simulink library "LibEEPROM_eeprom_example_ORIGINAL"  (Simulink 10.0)
settings: Solver=VariableStepAuto  StartTime=0.0  StopTime=10.0  RelTol=1e-3
undefined symbols (not defined in the file): CRC32_calc_and_EEPROM_Write_ALL, crc32_calc_intern, CRC32_EEPROM_Read, EEPROM_Mirror, EEPROM_Read, IO_Blk_Lib_TTC500, IO_EEPROM_GetStatus, IO_EEPROM_Init, IO_EEPROM_Write, Read_Mirror, Write_Mirror, Write_Mirror_prepare_EEPROM
libraries: simulink x56
(part 1 of 8)
settings Model: Creator=hokka  LastModifiedBy=hokka

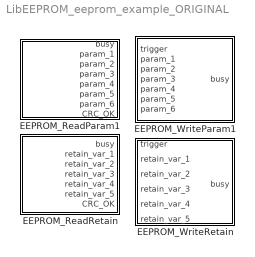
== system LibEEPROM_eeprom_example_ORIGINAL ==
  EEPROM_ReadParam1 : Subsystem  Priority=0  mask(Generated EEPROM_Read){}
      mask help: This Block was generated by the EEPROM Importer
      mask Help:
      | Read out the EEPROM for all given parameters and provide these values on the outports.
      | Reading is done at startup. As long as reading form EEPROM is not terminated for all parameters the busy flag will stay 'true'.
      | CRC_OK will be 0 as long as reading of EEPROM is not completed. Upon success the result is +1. If CRC check fails the result will be -1.
  EEPROM_ReadRetain : Subsystem  Priority=0  mask(Generated EEPROM_Read){}
      mask help: This Block was generated by the EEPROM Importer
      mask Help:
      | Read out the EEPROM for all given parameters and provide these values on the outports.
      | Reading is done at startup. As long as reading form EEPROM is not terminated for all parameters the busy flag will stay 'true'.
      | CRC_OK will be 0 as long as reading of EEPROM is not completed. Upon success the result is +1. If CRC check fails the result will be -1.
  EEPROM_WriteParam1 : Subsystem  Priority=0  mask(Generated EEPROM_Write){}
      mask help: This Block was generated by the EEPROM Importer
      mask Help:
      | Aufter receiving the positive edge of a trigger signal the EEPROM_Write - Block will store the parameters into the EEPROM together with the updated CRC32.
      | The busy flag will be 'true' as long as writing to EEPROM is not accomplished or any other EEPROM access is ongoing.
      | The busy flag needs not to be fed back as the trigger rise an internal pending activity as long as EEPROM is not accessible in order to accomplishe the actual writing as soon as the EEPROM is accessible again.
  EEPROM_WriteRetain : Subsystem  Priority=0  mask(Generated EEPROM_Write){}
      mask help: This Block was generated by the EEPROM Importer
      mask Help:
      | Aufter receiving the positive edge of a trigger signal the EEPROM_Write - Block will store the parameters into the EEPROM together with the updated CRC32.
      | The busy flag will be 'true' as long as writing to EEPROM is not accomplished or any other EEPROM access is ongoing.
      | The busy flag needs not to be fed back as the trigger rise an internal pending activity as long as EEPROM is not accessible in order to accomplishe the actual writing as soon as the EEPROM is accessible again.

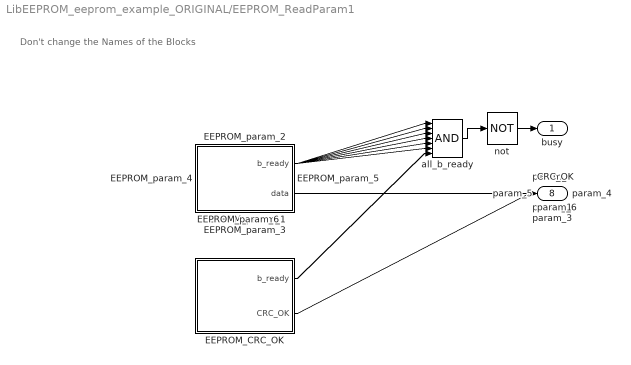
== system LibEEPROM_eeprom_example_ORIGINAL/EEPROM_ReadParam1 ==
  note: Don't change the Names of the Blocks
  EEPROM_CRC_OK : Subsystem  LoadFcn=|  mask(CRC32_EEPROM_Read_Code){SampleTime=-1, ttlib=IO_Blk_Lib_TTC500, ttDescription=CRC32_EEPROM_Read, tt_iolib_version=0.26, BasicAddr=4096, EndAddr=4110, offset=4111, length=4}
      | try
      | %
      | %Upgrade Information - standard BEGIN
      | new_color = 'blue';
      | new_ver = '0.26';
      | act_ver = get_param(gcb,'tt_iolib_version');
      | if not(strcmp(act_ver,new_ver))
      |     disp(['Upgrade block: ',gcb,char(10),'       Version: ',act_ver,' to ',new_ver]);
      |     %switch - case for specific upgrade information e.g. additional parameter required 
      |     %Change appearance and version information
      |     set_param(gcb,'ForegroundColor',new_color);
      |     set_param(gcb,'tt_iolib_version',new_ver);
      | end
      | %Upgrade Information - standard END
      | catch
      | %Standard catch section BEGIN
      | errordlg('An error occurred in a callback of the TTC580-BlockLib. Please open the Diagnostic Viewer for further details');
      | disp(' ');
      | disp('------------------------------------------------------------');
      | disp('An error occurred in a callback of the TTC580-BlockLib.');
      | disp(['Please check the parameters in the mask of ',gcb]);
      | disp('If you do not encounter any violations, then please '); 
      | disp('copy the following lines and report this to support@ttcontrol.com ');
      | disp('<< begin of error message dump >>');
      | disp(['Version of TTC580-BlockLib: ', get_param(gcb,'tt_iolib_version')]);
      | disp(get_param(gcb,'ttDescription'));
      | disp(gcb);
      | x=lasterror;disp(x.message);
      | disp(get_param(gcb,'MaskValues'));
      | disp(version);
      | disp(computer);
      | disp('<< end of error message dump >>');
      | disp('------------------------------------------------------------');
      | disp(' ');
      | %Standard catch section END
      | end
      mask help:
      | Calculate crc32 for the section [BasicAddr .. EndAddr] out of the EEPROM and compare to the content of a given address (=offset) in EEPROM.
      | The output CRC_OK may hold three possible values:
      | -1 => after EEPROM section was read, CRC check failed (terminal state)
      |   0 => reading of EEPROM section not completed yet, CRC check is pending
      | +1 => after EEPROM section was read, CRC check was successful (terminal state)
      mask init:
      | try
      | %%CT>
      | TAG_loc = get_param(gcb,'Tag');
      | if ~isempty(TAG_loc),[~,y]=regexp(TAG_loc,'(^[a-zA-Z0-9_]*)');
      |     if isempty(y) || y~=builtin('length',(TAG_loc)) %don't use length() alone!
      |         error(['The Tag: ',TAG_loc,' needs to start with a letter and may only contain the characters 0-9,a-Z,_ .']);
      | end,end
      | x=find_system(gcbh,'FollowLinks','on','LookUnderMasks','on','BlockType','S-Function');
      | for i=1:builtin('length',(x)) %don't use length() alone!
      |     set_param(x(i),'Tag',TAG_loc);
      | end
      | %<CT%
      | 
      | catch
      | %Standard catch section BEGIN
      | errordlg('An error occurred in a callback of the TTC580-BlockLib. Please open the Diagnostic Viewer for further details');
      | disp(' ');
      | disp('------------------------------------------------------------');
      | disp('An error occurred in a callback of the TTC580-BlockLib.');
      | disp(['Please check the parameters in the mask of ',gcb]);
      | disp('If you do not encounter any violations, then please '); 
      | disp('copy the following lines and report this to support@ttcontrol.com ');
      | disp('<< begin of error message dump >>');
      | disp(['Version of TTC580-BlockLib: ', get_param(gcb,'tt_iolib_version')]);
      | disp(get_param(gcb,'ttDescription'));
      | disp(gcb);
      | x=lasterror;disp(x.message);
      | disp(get_param(gcb,'MaskValues'));
      | disp(version);
      | disp(computer);
      | disp('<< end of error message dump >>');
      | disp('------------------------------------------------------------');
      | disp(' ');
      | %Standard catch section END
      | end
      settings: CopyFcn=%deleted
      mask Callback BasicAddr: %
      mask Callback EndAddr: %
      mask Callback offset: %
      mask Callback length: %
  EEPROM_param_1 : Subsystem  LoadFcn=|  mask(EEPROM_Read_Code){SampleTime=-1, ttlib=IO_Blk_Lib_TTC500, ttDescription=EEPROM_Read, tt_iolib_version=0.26, offset=4096, EEPROM_type=uint16}
      | try
      | %
      | %Upgrade Information - standard BEGIN
      | new_color = 'blue';
      | new_ver = '0.26';
      | act_ver = get_param(gcb,'tt_iolib_version');
      | if not(strcmp(act_ver,new_ver))
      |     disp(['Upgrade block: ',gcb,char(10),'       Version: ',act_ver,' to ',new_ver]);
      |     %switch - case for specific upgrade information e.g. additional parameter required 
      |     %Change appearance and version information
      |     set_param(gcb,'ForegroundColor',new_color);
      |     set_param(gcb,'tt_iolib_version',new_ver);
      | end
      | %Upgrade Information - standard END
      | catch
      | %Standard catch section BEGIN
      | errordlg('An error occurred in a callback of the TTC580-BlockLib. Please open the Diagnostic Viewer for further details');
      | disp(' ');
      | disp('------------------------------------------------------------');
      | disp('An error occurred in a callback of the TTC580-BlockLib.');
      | disp(['Please check the parameters in the mask of ',gcb]);
      | disp('If you do not encounter any violations, then please '); 
      | disp('copy the following lines and report this to support@ttcontrol.com ');
      | disp('<< begin of error message dump >>');
      | disp(['Version of TTC580-BlockLib: ', get_param(gcb,'tt_iolib_version')]);
      | disp(get_param(gcb,'ttDescription'));
      | disp(gcb);
      | x=lasterror;disp(x.message);
      | disp(get_param(gcb,'MaskValues'));
      | disp(version);
      | disp(computer);
      | disp('<< end of error message dump >>');
      | disp('------------------------------------------------------------');
      | disp(' ');
      | %Standard catch section END
      | end
      mask help:
      | Read data from the EEPROM.
      | Note that offset has to be in the range (0..65535 bytes)
      mask init:
      | try
      | switch EEPROM_type 
      |     case {'uint8'}
      |         length = 1; 
      |     case {'uint16'}; 
      |         length = 2; 
      |     case {'uint32'}
      |         length = 4; 
      |     case {'int8'}
      |         length = 1; 
      |     case {'int16'}; 
      |         length = 2; 
      |     case {'int32'}
      |         length = 4; 
      |     case {'single'}
      |         length = 4; 
      |     case {'double'}
      |         length = 8; 
      |     otherwise
      |         error('EEPROM_Read: unsupported type');
      | end
      | %%CT>
      | TAG_loc = get_param(gcb,'Tag');
      | if ~isempty(TAG_loc),[~,y]=regexp(TAG_loc,'(^[a-zA-Z0-9_]*)');
      |     if isempty(y) || y~=builtin('length',(TAG_loc)) %don't use length() alone!
      |         error(['The Tag: ',TAG_loc,' needs to start with a letter and may only contain the characters 0-9,a-Z,_ .']);
      | end,end
      | x=find_system(gcbh,'FollowLinks','on','LookUnderMasks','on','BlockType','S-Function');
      | for i=1:builtin('length',(x)) %don't use length() alone!
      |     set_param(x(i),'Tag',TAG_loc);
      | end
      | %<CT%
      | 
      | catch
      | %Standard catch section BEGIN
      | errordlg('An error occurred in a callback of the TTC580-BlockLib. Please open the Diagnostic Viewer for further details');
      | disp(' ');
      | disp('------------------------------------------------------------');
      | disp('An error occurred in a callback of the TTC580-BlockLib.');
      | disp(['Please check the parameters in the mask of ',gcb]);
      | disp('If you do not encounter any violations, then please '); 
      | disp('copy the following lines and report this to support@ttcontrol.com ');
      | disp('<< begin of error message dump >>');
      | disp(['Version of TTC580-BlockLib: ', get_param(gcb,'tt_iolib_version')]);
      | disp(get_param(gcb,'ttDescription'));
      | disp(gcb);
      | x=lasterror;disp(x.message);
      | disp(get_param(gcb,'MaskValues'));
      | disp(version);
      | disp(computer);
      | disp('<< end of error message dump >>');
      | disp('------------------------------------------------------------');
      | disp(' ');
      | %Standard catch section END
      | end
      settings: CopyFcn=%deleted
      mask Help: Parameter:<br>offset: [0..65535] place in the EEPROM where data shall be retieved from.<br>EEPROM_type: defines the length of data to be read from EEPROM. Possible values: uint8 (=1byte), uint16 (=2bytes), uint32 (=4bytes).<br><br>Output:<br>b_ready: when reading from EEPROM is not accomplished the output is FALSE.<br>data: Actual value that was retrieved from EEPROM.<br><br>Note: When the expression (offset + length) of Bytes exceed the limit of 65535 no  reading from EEPROM takes place and a constant zero is output as data and b_ready is FALSE.<br>When b_ready is not TRUE do not trust data as reading of EEPROM is not finished at startup of the ECU.<br><br>
      mask Callback offset: %
      mask TypeOptions EEPROM_type: uint8 | uint16 | uint32
      mask Callback EEPROM_type: %
  EEPROM_param_2 : Subsystem  LoadFcn=|  mask(EEPROM_Read_Code){SampleTime=-1, ttlib=IO_Blk_Lib_TTC500, ttDescription=EEPROM_Read, tt_iolib_version=0.26, offset=4098, EEPROM_type=uint16}
      | try
      | %
      | %Upgrade Information - standard BEGIN
      | new_color = 'blue';
      | new_ver = '0.26';
      | act_ver = get_param(gcb,'tt_iolib_version');
      | if not(strcmp(act_ver,new_ver))
      |     disp(['Upgrade block: ',gcb,char(10),'       Version: ',act_ver,' to ',new_ver]);
      |     %switch - case for specific upgrade information e.g. additional parameter required 
      |     %Change appearance and version information
      |     set_param(gcb,'ForegroundColor',new_color);
      |     set_param(gcb,'tt_iolib_version',new_ver);
      | end
      | %Upgrade Information - standard END
      | catch
      | %Standard catch section BEGIN
      | errordlg('An error occurred in a callback of the TTC580-BlockLib. Please open the Diagnostic Viewer for further details');
      | disp(' ');
      | disp('------------------------------------------------------------');
      | disp('An error occurred in a callback of the TTC580-BlockLib.');
      | disp(['Please check the parameters in the mask of ',gcb]);
      | disp('If you do not encounter any violations, then please '); 
      | disp('copy the following lines and report this to support@ttcontrol.com ');
      | disp('<< begin of error message dump >>');
      | disp(['Version of TTC580-BlockLib: ', get_param(gcb,'tt_iolib_version')]);
      | disp(get_param(gcb,'ttDescription'));
      | disp(gcb);
      | x=lasterror;disp(x.message);
      | disp(get_param(gcb,'MaskValues'));
      | disp(version);
      | disp(computer);
      | disp('<< end of error message dump >>');
      | disp('------------------------------------------------------------');
      | disp(' ');
      | %Standard catch section END
      | end
      mask help:
      | Read data from the EEPROM.
      | Note that offset has to be in the range (0..65535 bytes)
      mask init: same as LibEEPROM_eeprom_example_ORIGINAL/EEPROM_ReadParam1/EEPROM_param_1
      settings: CopyFcn=%deleted
      mask Help: Parameter:<br>offset: [0..65535] place in the EEPROM where data shall be retieved from.<br>EEPROM_type: defines the length of data to be read from EEPROM. Possible values: uint8 (=1byte), uint16 (=2bytes), uint32 (=4bytes).<br><br>Output:<br>b_ready: when reading from EEPROM is not accomplished the output is FALSE.<br>data: Actual value that was retrieved from EEPROM.<br><br>Note: When the expression (offset + length) of Bytes exceed the limit of 65535 no  reading from EEPROM takes place and a constant zero is output as data and b_ready is FALSE.<br>When b_ready is not TRUE do not trust data as reading of EEPROM is not finished at startup of the ECU.<br><br>
      mask Callback offset: %
      mask TypeOptions EEPROM_type: uint8 | uint16 | uint32
      mask Callback EEPROM_type: %
  EEPROM_param_3 : Subsystem  LoadFcn=|  mask(EEPROM_Read_Code){SampleTime=-1, ttlib=IO_Blk_Lib_TTC500, ttDescription=EEPROM_Read, tt_iolib_version=0.26, offset=4100, EEPROM_type=uint8}
      | try
      | %
      | %Upgrade Information - standard BEGIN
      | new_color = 'blue';
      | new_ver = '0.26';
      | act_ver = get_param(gcb,'tt_iolib_version');
      | if not(strcmp(act_ver,new_ver))
      |     disp(['Upgrade block: ',gcb,char(10),'       Version: ',act_ver,' to ',new_ver]);
      |     %switch - case for specific upgrade information e.g. additional parameter required 
      |     %Change appearance and version information
      |     set_param(gcb,'ForegroundColor',new_color);
      |     set_param(gcb,'tt_iolib_version',new_ver);
      | end
      | %Upgrade Information - standard END
      | catch
      | %Standard catch section BEGIN
      | errordlg('An error occurred in a callback of the TTC580-BlockLib. Please open the Diagnostic Viewer for further details');
      | disp(' ');
      | disp('------------------------------------------------------------');
      | disp('An error occurred in a callback of the TTC580-BlockLib.');
      | disp(['Please check the parameters in the mask of ',gcb]);
      | disp('If you do not encounter any violations, then please '); 
      | disp('copy the following lines and report this to support@ttcontrol.com ');
      | disp('<< begin of error message dump >>');
      | disp(['Version of TTC580-BlockLib: ', get_param(gcb,'tt_iolib_version')]);
      | disp(get_param(gcb,'ttDescription'));
      | disp(gcb);
      | x=lasterror;disp(x.message);
      | disp(get_param(gcb,'MaskValues'));
      | disp(version);
      | disp(computer);
      | disp('<< end of error message dump >>');
      | disp('------------------------------------------------------------');
      | disp(' ');
      | %Standard catch section END
      | end
      mask help:
      | Read data from the EEPROM.
      | Note that offset has to be in the range (0..65535 bytes)
      mask init: same as LibEEPROM_eeprom_example_ORIGINAL/EEPROM_ReadParam1/EEPROM_param_1
      settings: CopyFcn=%deleted
      mask Help: Parameter:<br>offset: [0..65535] place in the EEPROM where data shall be retieved from.<br>EEPROM_type: defines the length of data to be read from EEPROM. Possible values: uint8 (=1byte), uint16 (=2bytes), uint32 (=4bytes).<br><br>Output:<br>b_ready: when reading from EEPROM is not accomplished the output is FALSE.<br>data: Actual value that was retrieved from EEPROM.<br><br>Note: When the expression (offset + length) of Bytes exceed the limit of 65535 no  reading from EEPROM takes place and a constant zero is output as data and b_ready is FALSE.<br>When b_ready is not TRUE do not trust data as reading of EEPROM is not finished at startup of the ECU.<br><br>
      mask Callback offset: %
      mask TypeOptions EEPROM_type: uint8 | uint16 | uint32
      mask Callback EEPROM_type: %
  EEPROM_param_4 : Subsystem  LoadFcn=|  mask(EEPROM_Read_Code){SampleTime=-1, ttlib=IO_Blk_Lib_TTC500, ttDescription=EEPROM_Read, tt_iolib_version=0.26, offset=4101, EEPROM_type=uint32}
      | try
      | %
      | %Upgrade Information - standard BEGIN
      | new_color = 'blue';
      | new_ver = '0.26';
      | act_ver = get_param(gcb,'tt_iolib_version');
      | if not(strcmp(act_ver,new_ver))
      |     disp(['Upgrade block: ',gcb,char(10),'       Version: ',act_ver,' to ',new_ver]);
      |     %switch - case for specific upgrade information e.g. additional parameter required 
      |     %Change appearance and version information
      |     set_param(gcb,'ForegroundColor',new_color);
      |     set_param(gcb,'tt_iolib_version',new_ver);
      | end
      | %Upgrade Information - standard END
      | catch
      | %Standard catch section BEGIN
      | errordlg('An error occurred in a callback of the TTC580-BlockLib. Please open the Diagnostic Viewer for further details');
      | disp(' ');
      | disp('------------------------------------------------------------');
      | disp('An error occurred in a callback of the TTC580-BlockLib.');
      | disp(['Please check the parameters in the mask of ',gcb]);
      | disp('If you do not encounter any violations, then please '); 
      | disp('copy the following lines and report this to support@ttcontrol.com ');
      | disp('<< begin of error message dump >>');
      | disp(['Version of TTC580-BlockLib: ', get_param(gcb,'tt_iolib_version')]);
      | disp(get_param(gcb,'ttDescription'));
      | disp(gcb);
      | x=lasterror;disp(x.message);
      | disp(get_param(gcb,'MaskValues'));
      | disp(version);
      | disp(computer);
      | disp('<< end of error message dump >>');
      | disp('------------------------------------------------------------');
      | disp(' ');
      | %Standard catch section END
      | end
      mask help:
      | Read data from the EEPROM.
      | Note that offset has to be in the range (0..65535 bytes)
      mask init: same as LibEEPROM_eeprom_example_ORIGINAL/EEPROM_ReadParam1/EEPROM_param_1
      settings: CopyFcn=%deleted
      mask Help: Parameter:<br>offset: [0..65535] place in the EEPROM where data shall be retieved from.<br>EEPROM_type: defines the length of data to be read from EEPROM. Possible values: uint8 (=1byte), uint16 (=2bytes), uint32 (=4bytes).<br><br>Output:<br>b_ready: when reading from EEPROM is not accomplished the output is FALSE.<br>data: Actual value that was retrieved from EEPROM.<br><br>Note: When the expression (offset + length) of Bytes exceed the limit of 65535 no  reading from EEPROM takes place and a constant zero is output as data and b_ready is FALSE.<br>When b_ready is not TRUE do not trust data as reading of EEPROM is not finished at startup of the ECU.<br><br>
      mask Callback offset: %
      mask TypeOptions EEPROM_type: uint8 | uint16 | uint32
      mask Callback EEPROM_type: %
  EEPROM_param_5 : Subsystem  LoadFcn=|  mask(EEPROM_Read_Code){SampleTime=-1, ttlib=IO_Blk_Lib_TTC500, ttDescription=EEPROM_Read, tt_iolib_version=0.26, offset=4105, EEPROM_type=uint32}
      | try
      | %
      | %Upgrade Information - standard BEGIN
      | new_color = 'blue';
      | new_ver = '0.26';
      | act_ver = get_param(gcb,'tt_iolib_version');
      | if not(strcmp(act_ver,new_ver))
      |     disp(['Upgrade block: ',gcb,char(10),'       Version: ',act_ver,' to ',new_ver]);
      |     %switch - case for specific upgrade information e.g. additional parameter required 
      |     %Change appearance and version information
      |     set_param(gcb,'ForegroundColor',new_color);
      |     set_param(gcb,'tt_iolib_version',new_ver);
      | end
      | %Upgrade Information - standard END
      | catch
      | %Standard catch section BEGIN
      | errordlg('An error occurred in a callback of the TTC580-BlockLib. Please open the Diagnostic Viewer for further details');
      | disp(' ');
      | disp('------------------------------------------------------------');
      | disp('An error occurred in a callback of the TTC580-BlockLib.');
      | disp(['Please check the parameters in the mask of ',gcb]);
      | disp('If you do not encounter any violations, then please '); 
      | disp('copy the following lines and report this to support@ttcontrol.com ');
      | disp('<< begin of error message dump >>');
      | disp(['Version of TTC580-BlockLib: ', get_param(gcb,'tt_iolib_version')]);
      | disp(get_param(gcb,'ttDescription'));
      | disp(gcb);
      | x=lasterror;disp(x.message);
      | disp(get_param(gcb,'MaskValues'));
      | disp(version);
      | disp(computer);
      | disp('<< end of error message dump >>');
      | disp('------------------------------------------------------------');
      | disp(' ');
      | %Standard catch section END
      | end
      mask help:
      | Read data from the EEPROM.
      | Note that offset has to be in the range (0..65535 bytes)
      mask init: same as LibEEPROM_eeprom_example_ORIGINAL/EEPROM_ReadParam1/EEPROM_param_1
      settings: CopyFcn=%deleted
      mask Help: Parameter:<br>offset: [0..65535] place in the EEPROM where data shall be retieved from.<br>EEPROM_type: defines the length of data to be read from EEPROM. Possible values: uint8 (=1byte), uint16 (=2bytes), uint32 (=4bytes).<br><br>Output:<br>b_ready: when reading from EEPROM is not accomplished the output is FALSE.<br>data: Actual value that was retrieved from EEPROM.<br><br>Note: When the expression (offset + length) of Bytes exceed the limit of 65535 no  reading from EEPROM takes place and a constant zero is output as data and b_ready is FALSE.<br>When b_ready is not TRUE do not trust data as reading of EEPROM is not finished at startup of the ECU.<br><br>
      mask Callback offset: %
      mask TypeOptions EEPROM_type: uint8 | uint16 | uint32
      mask Callback EEPROM_type: %
  EEPROM_param_6 : Subsystem  LoadFcn=|  mask(EEPROM_Read_Code){SampleTime=-1, ttlib=IO_Blk_Lib_TTC500, ttDescription=EEPROM_Read, tt_iolib_version=0.26, offset=4109, EEPROM_type=uint16}
      | try
      | %
      | %Upgrade Information - standard BEGIN
      | new_color = 'blue';
      | new_ver = '0.26';
      | act_ver = get_param(gcb,'tt_iolib_version');
      | if not(strcmp(act_ver,new_ver))
      |     disp(['Upgrade block: ',gcb,char(10),'       Version: ',act_ver,' to ',new_ver]);
      |     %switch - case for specific upgrade information e.g. additional parameter required 
      |     %Change appearance and version information
      |     set_param(gcb,'ForegroundColor',new_color);
      |     set_param(gcb,'tt_iolib_version',new_ver);
      | end
      | %Upgrade Information - standard END
      | catch
      | %Standard catch section BEGIN
      | errordlg('An error occurred in a callback of the TTC580-BlockLib. Please open the Diagnostic Viewer for further details');
      | disp(' ');
      | disp('------------------------------------------------------------');
      | disp('An error occurred in a callback of the TTC580-BlockLib.');
      | disp(['Please check the parameters in the mask of ',gcb]);
      | disp('If you do not encounter any violations, then please '); 
      | disp('copy the following lines and report this to support@ttcontrol.com ');
      | disp('<< begin of error message dump >>');
      | disp(['Version of TTC580-BlockLib: ', get_param(gcb,'tt_iolib_version')]);
      | disp(get_param(gcb,'ttDescription'));
      | disp(gcb);
      | x=lasterror;disp(x.message);
      | disp(get_param(gcb,'MaskValues'));
      | disp(version);
      | disp(computer);
      | disp('<< end of error message dump >>');
      | disp('------------------------------------------------------------');
      | disp(' ');
      | %Standard catch section END
      | end
      mask help:
      | Read data from the EEPROM.
      | Note that offset has to be in the range (0..65535 bytes)
      mask init: same as LibEEPROM_eeprom_example_ORIGINAL/EEPROM_ReadParam1/EEPROM_param_1
      settings: CopyFcn=%deleted
      mask Help: Parameter:<br>offset: [0..65535] place in the EEPROM where data shall be retieved from.<br>EEPROM_type: defines the length of data to be read from EEPROM. Possible values: uint8 (=1byte), uint16 (=2bytes), uint32 (=4bytes).<br><br>Output:<br>b_ready: when reading from EEPROM is not accomplished the output is FALSE.<br>data: Actual value that was retrieved from EEPROM.<br><br>Note: When the expression (offset + length) of Bytes exceed the limit of 65535 no  reading from EEPROM takes place and a constant zero is output as data and b_ready is FALSE.<br>When b_ready is not TRUE do not trust data as reading of EEPROM is not finished at startup of the ECU.<br><br>
      mask Callback offset: %
      mask TypeOptions EEPROM_type: uint8 | uint16 | uint32
      mask Callback EEPROM_type: %
  all_b_ready : Logic  Inputs=7  AllPortsSameDT=off  OutDataTypeStr=boolean
  not : Logic  Operator=NOT  Inputs=1  AllPortsSameDT=off  OutDataTypeStr=boolean
  busy : Outport  VectorParamsAs1DForOutWhenUnconnected=off
  param_1 : Outport  Port=2  VectorParamsAs1DForOutWhenUnconnected=off
  param_2 : Outport  Port=3  VectorParamsAs1DForOutWhenUnconnected=off
  param_3 : Outport  Port=4  VectorParamsAs1DForOutWhenUnconnected=off
  param_4 : Outport  Port=5  VectorParamsAs1DForOutWhenUnconnected=off
  param_5 : Outport  Port=6  VectorParamsAs1DForOutWhenUnconnected=off
  param_6 : Outport  Port=7  VectorParamsAs1DForOutWhenUnconnected=off
  CRC_OK : Outport  Port=8  VectorParamsAs1DForOutWhenUnconnected=off
  wires:
  not/1 -> busy/1
  all_b_ready/1 -> not/1
  EEPROM_param_1/1(b_ready) -> all_b_ready/1
  EEPROM_param_1/2(data) -> param_1/1
  EEPROM_param_2/1(b_ready) -> all_b_ready/2
  EEPROM_param_2/2(data) -> param_2/1
  EEPROM_param_3/1(b_ready) -> all_b_ready/3
  EEPROM_param_3/2(data) -> param_3/1
  EEPROM_param_4/1(b_ready) -> all_b_ready/4
  EEPROM_param_4/2(data) -> param_4/1
  EEPROM_param_5/1(b_ready) -> all_b_ready/5
  EEPROM_param_5/2(data) -> param_5/1
  EEPROM_param_6/1(b_ready) -> all_b_ready/6
  EEPROM_param_6/2(data) -> param_6/1
  EEPROM_CRC_OK/1(b_ready) -> all_b_ready/7
  EEPROM_CRC_OK/2(CRC_OK) -> CRC_OK/1

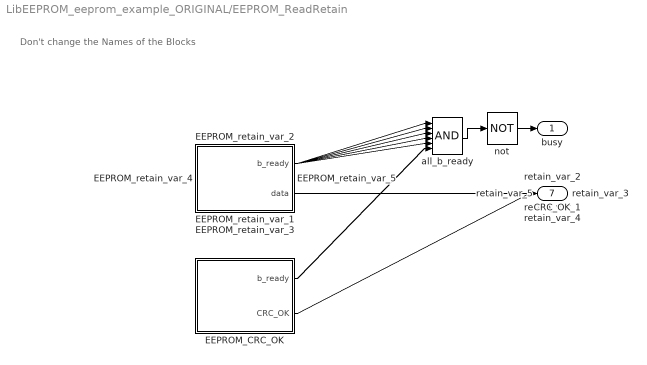
== system LibEEPROM_eeprom_example_ORIGINAL/EEPROM_ReadRetain ==
  note: Don't change the Names of the Blocks
  EEPROM_CRC_OK : Subsystem  LoadFcn=|  mask(CRC32_EEPROM_Read_Code){SampleTime=-1, ttlib=IO_Blk_Lib_TTC500, ttDescription=CRC32_EEPROM_Read, tt_iolib_version=0.26, BasicAddr=8192, EndAddr=8199, offset=8200, length=4}
      | try
      | %
      | %Upgrade Information - standard BEGIN
      | new_color = 'blue';
      | new_ver = '0.26';
      | act_ver = get_param(gcb,'tt_iolib_version');
      | if not(strcmp(act_ver,new_ver))
      |     disp(['Upgrade block: ',gcb,char(10),'       Version: ',act_ver,' to ',new_ver]);
      |     %switch - case for specific upgrade information e.g. additional parameter required 
      |     %Change appearance and version information
      |     set_param(gcb,'ForegroundColor',new_color);
      |     set_param(gcb,'tt_iolib_version',new_ver);
      | end
      | %Upgrade Information - standard END
      | catch
      | %Standard catch section BEGIN
      | errordlg('An error occurred in a callback of the TTC580-BlockLib. Please open the Diagnostic Viewer for further details');
      | disp(' ');
      | disp('------------------------------------------------------------');
      | disp('An error occurred in a callback of the TTC580-BlockLib.');
      | disp(['Please check the parameters in the mask of ',gcb]);
      | disp('If you do not encounter any violations, then please '); 
      | disp('copy the following lines and report this to support@ttcontrol.com ');
      | disp('<< begin of error message dump >>');
      | disp(['Version of TTC580-BlockLib: ', get_param(gcb,'tt_iolib_version')]);
      | disp(get_param(gcb,'ttDescription'));
      | disp(gcb);
      | x=lasterror;disp(x.message);
      | disp(get_param(gcb,'MaskValues'));
      | disp(version);
      | disp(computer);
      | disp('<< end of error message dump >>');
      | disp('------------------------------------------------------------');
      | disp(' ');
      | %Standard catch section END
      | end
      mask help:
      | Calculate crc32 for the section [BasicAddr .. EndAddr] out of the EEPROM and compare to the content of a given address (=offset) in EEPROM.
      | The output CRC_OK may hold three possible values:
      | -1 => after EEPROM section was read, CRC check failed (terminal state)
      |   0 => reading of EEPROM section not completed yet, CRC check is pending
      | +1 => after EEPROM section was read, CRC check was successful (terminal state)
      mask init: same as LibEEPROM_eeprom_example_ORIGINAL/EEPROM_ReadParam1/EEPROM_CRC_OK
      settings: CopyFcn=%deleted
      mask Callback BasicAddr: %
      mask Callback EndAddr: %
      mask Callback offset: %
      mask Callback length: %
  EEPROM_retain_var_1 : Subsystem  LoadFcn=|  mask(EEPROM_Read_Code){SampleTime=-1, ttlib=IO_Blk_Lib_TTC500, ttDescription=EEPROM_Read, tt_iolib_version=0.26, offset=8192, EEPROM_type=uint16}
      | try
      | %
      | %Upgrade Information - standard BEGIN
      | new_color = 'blue';
      | new_ver = '0.26';
      | act_ver = get_param(gcb,'tt_iolib_version');
      | if not(strcmp(act_ver,new_ver))
      |     disp(['Upgrade block: ',gcb,char(10),'       Version: ',act_ver,' to ',new_ver]);
      |     %switch - case for specific upgrade information e.g. additional parameter required 
      |     %Change appearance and version information
      |     set_param(gcb,'ForegroundColor',new_color);
      |     set_param(gcb,'tt_iolib_version',new_ver);
      | end
      | %Upgrade Information - standard END
      | catch
      | %Standard catch section BEGIN
      | errordlg('An error occurred in a callback of the TTC580-BlockLib. Please open the Diagnostic Viewer for further details');
      | disp(' ');
      | disp('------------------------------------------------------------');
      | disp('An error occurred in a callback of the TTC580-BlockLib.');
      | disp(['Please check the parameters in the mask of ',gcb]);
      | disp('If you do not encounter any violations, then please '); 
      | disp('copy the following lines and report this to support@ttcontrol.com ');
      | disp('<< begin of error message dump >>');
      | disp(['Version of TTC580-BlockLib: ', get_param(gcb,'tt_iolib_version')]);
      | disp(get_param(gcb,'ttDescription'));
      | disp(gcb);
      | x=lasterror;disp(x.message);
      | disp(get_param(gcb,'MaskValues'));
      | disp(version);
      | disp(computer);
      | disp('<< end of error message dump >>');
      | disp('------------------------------------------------------------');
      | disp(' ');
      | %Standard catch section END
      | end
      mask help:
      | Read data from the EEPROM.
      | Note that offset has to be in the range (0..65535 bytes)
      mask init: same as LibEEPROM_eeprom_example_ORIGINAL/EEPROM_ReadParam1/EEPROM_param_1
      settings: CopyFcn=%deleted
      mask Help: Parameter:<br>offset: [0..65535] place in the EEPROM where data shall be retieved from.<br>EEPROM_type: defines the length of data to be read from EEPROM. Possible values: uint8 (=1byte), uint16 (=2bytes), uint32 (=4bytes).<br><br>Output:<br>b_ready: when reading from EEPROM is not accomplished the output is FALSE.<br>data: Actual value that was retrieved from EEPROM.<br><br>Note: When the expression (offset + length) of Bytes exceed the limit of 65535 no  reading from EEPROM takes place and a constant zero is output as data and b_ready is FALSE.<br>When b_ready is not TRUE do not trust data as reading of EEPROM is not finished at startup of the ECU.<br><br>
      mask Callback offset: %
      mask TypeOptions EEPROM_type: uint8 | uint16 | uint32
      mask Callback EEPROM_type: %
  EEPROM_retain_var_2 : Subsystem  LoadFcn=|  mask(EEPROM_Read_Code){SampleTime=-1, ttlib=IO_Blk_Lib_TTC500, ttDescription=EEPROM_Read, tt_iolib_version=0.26, offset=8194, EEPROM_type=uint8}
      | try
      | %
      | %Upgrade Information - standard BEGIN
      | new_color = 'blue';
      | new_ver = '0.26';
      | act_ver = get_param(gcb,'tt_iolib_version');
      | if not(strcmp(act_ver,new_ver))
      |     disp(['Upgrade block: ',gcb,char(10),'       Version: ',act_ver,' to ',new_ver]);
      |     %switch - case for specific upgrade information e.g. additional parameter required 
      |     %Change appearance and version information
      |     set_param(gcb,'ForegroundColor',new_color);
      |     set_param(gcb,'tt_iolib_version',new_ver);
      | end
      | %Upgrade Information - standard END
      | catch
      | %Standard catch section BEGIN
      | errordlg('An error occurred in a callback of the TTC580-BlockLib. Please open the Diagnostic Viewer for further details');
      | disp(' ');
      | disp('------------------------------------------------------------');
      | disp('An error occurred in a callback of the TTC580-BlockLib.');
      | disp(['Please check the parameters in the mask of ',gcb]);
      | disp('If you do not encounter any violations, then please '); 
      | disp('copy the following lines and report this to support@ttcontrol.com ');
      | disp('<< begin of error message dump >>');
      | disp(['Version of TTC580-BlockLib: ', get_param(gcb,'tt_iolib_version')]);
      | disp(get_param(gcb,'ttDescription'));
      | disp(gcb);
      | x=lasterror;disp(x.message);
      | disp(get_param(gcb,'MaskValues'));
      | disp(version);
      | disp(computer);
      | disp('<< end of error message dump >>');
      | disp('------------------------------------------------------------');
      | disp(' ');
      | %Standard catch section END
      | end
      mask help:
      | Read data from the EEPROM.
      | Note that offset has to be in the range (0..65535 bytes)
      mask init: same as LibEEPROM_eeprom_example_ORIGINAL/EEPROM_ReadParam1/EEPROM_param_1
      settings: CopyFcn=%deleted
      mask Help: Parameter:<br>offset: [0..65535] place in the EEPROM where data shall be retieved from.<br>EEPROM_type: defines the length of data to be read from EEPROM. Possible values: uint8 (=1byte), uint16 (=2bytes), uint32 (=4bytes).<br><br>Output:<br>b_ready: when reading from EEPROM is not accomplished the output is FALSE.<br>data: Actual value that was retrieved from EEPROM.<br><br>Note: When the expression (offset + length) of Bytes exceed the limit of 65535 no  reading from EEPROM takes place and a constant zero is output as data and b_ready is FALSE.<br>When b_ready is not TRUE do not trust data as reading of EEPROM is not finished at startup of the ECU.<br><br>
      mask Callback offset: %
      mask TypeOptions EEPROM_type: uint8 | uint16 | uint32
      mask Callback EEPROM_type: %
  EEPROM_retain_var_3 : Subsystem  LoadFcn=|  mask(EEPROM_Read_Code){SampleTime=-1, ttlib=IO_Blk_Lib_TTC500, ttDescription=EEPROM_Read, tt_iolib_version=0.26, offset=8195, EEPROM_type=uint8}
      | try
      | %
      | %Upgrade Information - standard BEGIN
      | new_color = 'blue';
      | new_ver = '0.26';
      | act_ver = get_param(gcb,'tt_iolib_version');
      | if not(strcmp(act_ver,new_ver))
      |     disp(['Upgrade block: ',gcb,char(10),'       Version: ',act_ver,' to ',new_ver]);
      |     %switch - case for specific upgrade information e.g. additional parameter required 
      |     %Change appearance and version information
      |     set_param(gcb,'ForegroundColor',new_color);
      |     set_param(gcb,'tt_iolib_version',new_ver);
      | end
      | %Upgrade Information - standard END
      | catch
      | %Standard catch section BEGIN
      | errordlg('An error occurred in a callback of the TTC580-BlockLib. Please open the Diagnostic Viewer for further details');
      | disp(' ');
      | disp('------------------------------------------------------------');
      | disp('An error occurred in a callback of the TTC580-BlockLib.');
      | disp(['Please check the parameters in the mask of ',gcb]);
      | disp('If you do not encounter any violations, then please '); 
      | disp('copy the following lines and report this to support@ttcontrol.com ');
      | disp('<< begin of error message dump >>');
      | disp(['Version of TTC580-BlockLib: ', get_param(gcb,'tt_iolib_version')]);
      | disp(get_param(gcb,'ttDescription'));
      | disp(gcb);
      | x=lasterror;disp(x.message);
      | disp(get_param(gcb,'MaskValues'));
      | disp(version);
      | disp(computer);
      | disp('<< end of error message dump >>');
      | disp('------------------------------------------------------------');
      | disp(' ');
      | %Standard catch section END
      | end
      mask help:
      | Read data from the EEPROM.
      | Note that offset has to be in the range (0..65535 bytes)
      mask init: same as LibEEPROM_eeprom_example_ORIGINAL/EEPROM_ReadParam1/EEPROM_param_1
      settings: CopyFcn=%deleted
      mask Help: Parameter:<br>offset: [0..65535] place in the EEPROM where data shall be retieved from.<br>EEPROM_type: defines the length of data to be read from EEPROM. Possible values: uint8 (=1byte), uint16 (=2bytes), uint32 (=4bytes).<br><br>Output:<br>b_ready: when reading from EEPROM is not accomplished the output is FALSE.<br>data: Actual value that was retrieved from EEPROM.<br><br>Note: When the expression (offset + length) of Bytes exceed the limit of 65535 no  reading from EEPROM takes place and a constant zero is output as data and b_ready is FALSE.<br>When b_ready is not TRUE do not trust data as reading of EEPROM is not finished at startup of the ECU.<br><br>
      mask Callback offset: %
      mask TypeOptions EEPROM_type: uint8 | uint16 | uint32
      mask Callback EEPROM_type: %
  EEPROM_retain_var_4 : Subsystem  LoadFcn=|  mask(EEPROM_Read_Code){SampleTime=-1, ttlib=IO_Blk_Lib_TTC500, ttDescription=EEPROM_Read, tt_iolib_version=0.26, offset=8196, EEPROM_type=uint16}
      | try
      | %
      | %Upgrade Information - standard BEGIN
      | new_color = 'blue';
      | new_ver = '0.26';
      | act_ver = get_param(gcb,'tt_iolib_version');
      | if not(strcmp(act_ver,new_ver))
      |     disp(['Upgrade block: ',gcb,char(10),'       Version: ',act_ver,' to ',new_ver]);
      |     %switch - case for specific upgrade information e.g. additional parameter required 
      |     %Change appearance and version information
      |     set_param(gcb,'ForegroundColor',new_color);
      |     set_param(gcb,'tt_iolib_version',new_ver);
      | end
      | %Upgrade Information - standard END
      | catch
      | %Standard catch section BEGIN
      | errordlg('An error occurred in a callback of the TTC580-BlockLib. Please open the Diagnostic Viewer for further details');
      | disp(' ');
      | disp('------------------------------------------------------------');
      | disp('An error occurred in a callback of the TTC580-BlockLib.');
      | disp(['Please check the parameters in the mask of ',gcb]);
      | disp('If you do not encounter any violations, then please '); 
      | disp('copy the following lines and report this to support@ttcontrol.com ');
      | disp('<< begin of error message dump >>');
      | disp(['Version of TTC580-BlockLib: ', get_param(gcb,'tt_iolib_version')]);
      | disp(get_param(gcb,'ttDescription'));
      | disp(gcb);
      | x=lasterror;disp(x.message);
      | disp(get_param(gcb,'MaskValues'));
      | disp(version);
      | disp(computer);
      | disp('<< end of error message dump >>');
      | disp('------------------------------------------------------------');
      | disp(' ');
      | %Standard catch section END
      | end
      mask help:
      | Read data from the EEPROM.
      | Note that offset has to be in the range (0..65535 bytes)
      mask init: same as LibEEPROM_eeprom_example_ORIGINAL/EEPROM_ReadParam1/EEPROM_param_1
      settings: CopyFcn=%deleted
      mask Help: Parameter:<br>offset: [0..65535] place in the EEPROM where data shall be retieved from.<br>EEPROM_type: defines the length of data to be read from EEPROM. Possible values: uint8 (=1byte), uint16 (=2bytes), uint32 (=4bytes).<br><br>Output:<br>b_ready: when reading from EEPROM is not accomplished the output is FALSE.<br>data: Actual value that was retrieved from EEPROM.<br><br>Note: When the expression (offset + length) of Bytes exceed the limit of 65535 no  reading from EEPROM takes place and a constant zero is output as data and b_ready is FALSE.<br>When b_ready is not TRUE do not trust data as reading of EEPROM is not finished at startup of the ECU.<br><br>
      mask Callback offset: %
      mask TypeOptions EEPROM_type: uint8 | uint16 | uint32
      mask Callback EEPROM_type: %
  EEPROM_retain_var_5 : Subsystem  LoadFcn=|  mask(EEPROM_Read_Code){SampleTime=-1, ttlib=IO_Blk_Lib_TTC500, ttDescription=EEPROM_Read, tt_iolib_version=0.26, offset=8198, EEPROM_type=uint16}
      | try
      | %
      | %Upgrade Information - standard BEGIN
      | new_color = 'blue';
      | new_ver = '0.26';
      | act_ver = get_param(gcb,'tt_iolib_version');
      | if not(strcmp(act_ver,new_ver))
      |     disp(['Upgrade block: ',gcb,char(10),'       Version: ',act_ver,' to ',new_ver]);
      |     %switch - case for specific upgrade information e.g. additional parameter required 
      |     %Change appearance and version information
      |     set_param(gcb,'ForegroundColor',new_color);
      |     set_param(gcb,'tt_iolib_version',new_ver);
      | end
      | %Upgrade Information - standard END
      | catch
      | %Standard catch section BEGIN
      | errordlg('An error occurred in a callback of the TTC580-BlockLib. Please open the Diagnostic Viewer for further details');
      | disp(' ');
      | disp('------------------------------------------------------------');
      | disp('An error occurred in a callback of the TTC580-BlockLib.');
      | disp(['Please check the parameters in the mask of ',gcb]);
      | disp('If you do not encounter any violations, then please '); 
      | disp('copy the following lines and report this to support@ttcontrol.com ');
      | disp('<< begin of error message dump >>');
      | disp(['Version of TTC580-BlockLib: ', get_param(gcb,'tt_iolib_version')]);
      | disp(get_param(gcb,'ttDescription'));
      | disp(gcb);
      | x=lasterror;disp(x.message);
      | disp(get_param(gcb,'MaskValues'));
      | disp(version);
      | disp(computer);
      | disp('<< end of error message dump >>');
      | disp('------------------------------------------------------------');
      | disp(' ');
      | %Standard catch section END
      | end
      mask help:
      | Read data from the EEPROM.
      | Note that offset has to be in the range (0..65535 bytes)
      mask init: same as LibEEPROM_eeprom_example_ORIGINAL/EEPROM_ReadParam1/EEPROM_param_1
      settings: CopyFcn=%deleted
      mask Help: Parameter:<br>offset: [0..65535] place in the EEPROM where data shall be retieved from.<br>EEPROM_type: defines the length of data to be read from EEPROM. Possible values: uint8 (=1byte), uint16 (=2bytes), uint32 (=4bytes).<br><br>Output:<br>b_ready: when reading from EEPROM is not accomplished the output is FALSE.<br>data: Actual value that was retrieved from EEPROM.<br><br>Note: When the expression (offset + length) of Bytes exceed the limit of 65535 no  reading from EEPROM takes place and a constant zero is output as data and b_ready is FALSE.<br>When b_ready is not TRUE do not trust data as reading of EEPROM is not finished at startup of the ECU.<br><br>
      mask Callback offset: %
      mask TypeOptions EEPROM_type: uint8 | uint16 | uint32
      mask Callback EEPROM_type: %
  all_b_ready : Logic  Inputs=6  AllPortsSameDT=off  OutDataTypeStr=boolean
  not : Logic  Operator=NOT  Inputs=1  AllPortsSameDT=off  OutDataTypeStr=boolean
  busy : Outport  VectorParamsAs1DForOutWhenUnconnected=off
  retain_var_1 : Outport  Port=2  VectorParamsAs1DForOutWhenUnconnected=off
  retain_var_2 : Outport  Port=3  VectorParamsAs1DForOutWhenUnconnected=off
  retain_var_3 : Outport  Port=4  VectorParamsAs1DForOutWhenUnconnected=off
  retain_var_4 : Outport  Port=5  VectorParamsAs1DForOutWhenUnconnected=off
  retain_var_5 : Outport  Port=6  VectorParamsAs1DForOutWhenUnconnected=off
  CRC_OK : Outport  Port=7  VectorParamsAs1DForOutWhenUnconnected=off
  wires:
  not/1 -> busy/1
  all_b_ready/1 -> not/1
  EEPROM_retain_var_1/1(b_ready) -> all_b_ready/1
  EEPROM_retain_var_1/2(data) -> retain_var_1/1
  EEPROM_retain_var_2/1(b_ready) -> all_b_ready/2
  EEPROM_retain_var_2/2(data) -> retain_var_2/1
  EEPROM_retain_var_3/1(b_ready) -> all_b_ready/3
  EEPROM_retain_var_3/2(data) -> retain_var_3/1
  EEPROM_retain_var_4/1(b_ready) -> all_b_ready/4
  EEPROM_retain_var_4/2(data) -> retain_var_4/1
  EEPROM_retain_var_5/1(b_ready) -> all_b_ready/5
  EEPROM_retain_var_5/2(data) -> retain_var_5/1
  EEPROM_CRC_OK/1(b_ready) -> all_b_ready/6
  EEPROM_CRC_OK/2(CRC_OK) -> CRC_OK/1
